simulink model "ControlePD_ind"  (R2020a)
settings: Solver=FixedStepAuto  StartTime=0.0  StopTime=10.0  FixedStep=Ts
values from neighbouring files (symbols this model uses):
  Beff = 50    [Ex4.m]
  Jeff = 2.2    [Ex4.m]
  K = 17.7    [Ex4.m]
  Kd = (2*qsi*wn*Jeff - Beff)/K    (= -0.338983050847)    [Ex4.m]
  Kp = (wn^2*Jeff)/K    (= 12.4293785311)    [Ex4.m]
  N = 10    [Ex4.m]
  r = 1    [Ex4.m]
  SP_theta = [60;-110;20;20;20]    [Ex4.m]
(part 3 of 3)

== matlab function ControlePD_ind/Perturbação/MATLAB Function4 ==
  data: M input; V input; tau5 output; G input; ddth1 input; ddth2 input; ddth3 input; ddth4 input; ddth5 input
function tau5  = calcul_dk5(M, V, G,ddth1,ddth2,ddth3,ddth4,ddth5)

ddth = [ddth1; ddth2; ddth3; ddth4; ddth5];
tau5 = M(5,:)*ddth + V(5,1) + G(5);
